simulink model "motor_channel"  (R2021a)
settings: configuration reference "motor_ctrl_config" (kept outside this file)
model workspace (MAT data in the model file):
  debounce_cnt = Simulink.Parameter
  debounce_cnt.Value = 4
  debounce_cnt.DataType = 'int16'
  debounce_cnt.Dimensions = [1 1]
  long_cnt = Simulink.Parameter
  long_cnt.Value = 6000
  long_cnt.DataType = 'int16'
  long_cnt.Dimensions = [1 1]
  longpress_cnt = Simulink.Parameter
  longpress_cnt.Value = 100
  longpress_cnt.DataType = 'int16'
  longpress_cnt.Dimensions = [1 1]
  short_cnt = Simulink.Parameter
  short_cnt.Value = 20
  short_cnt.DataType = 'int16'
  short_cnt.Dimensions = [1 1]
  transfer_cnt = Simulink.Parameter
  transfer_cnt.Value = 50
  transfer_cnt.DataType = 'int16'
  transfer_cnt.Dimensions = [1 1]
settings Model: DataDictionary=motor_ctrl_data.sldd  ParameterArgumentNames=debounce_cnt,long_cnt,longpress_cnt,short_cnt,transfer_cnt  OrderedModelArguments=off  Creator=Litao  LastModifiedBy=Litao
settings ConfigSetRef: SourceName=motor_ctrl_config

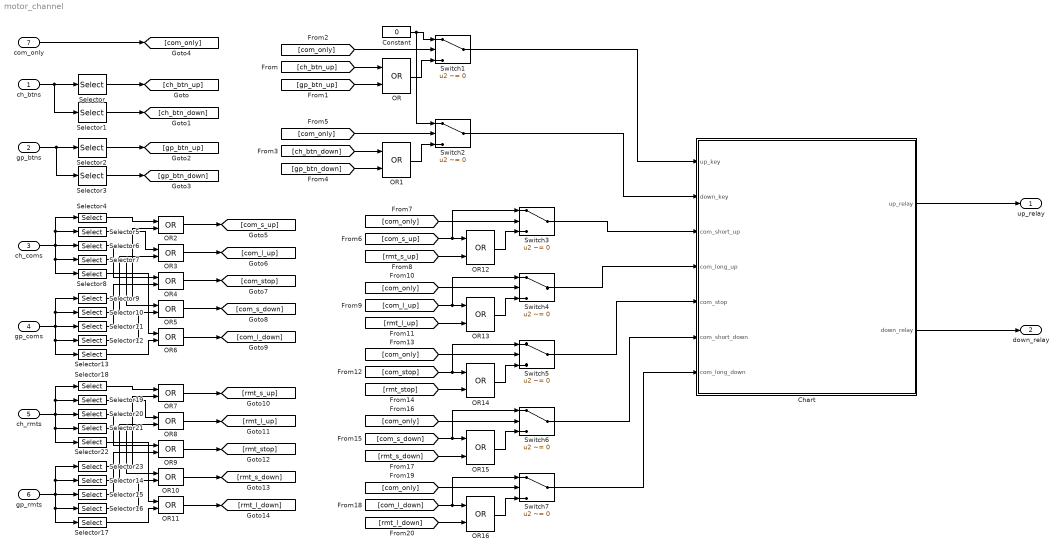
== system motor_channel ==
  ch_btns : Inport  OutMin=0  OutMax=1  OutDataTypeStr=int16  PortDimensions=2
  gp_btns : Inport  Port=2  OutMin=0  OutMax=1  OutDataTypeStr=int16  PortDimensions=2
  ch_coms : Inport  Port=3  OutMin=0  OutMax=1  OutDataTypeStr=int16  PortDimensions=5
  gp_coms : Inport  Port=4  OutMin=0  OutMax=1  OutDataTypeStr=int16  PortDimensions=5
  ch_rmts : Inport  Port=5  OutMin=0  OutMax=1  OutDataTypeStr=int16  PortDimensions=5
  gp_rmts : Inport  Port=6  OutMin=0  OutMax=1  OutDataTypeStr=int16  PortDimensions=5
  com_only : Inport  Port=7  OutMin=0  OutMax=1  OutDataTypeStr=int16  PortDimensions=1
  Chart : Stateflow chart
      settings: PortSchema="{\"entries\":[{\"content\":{\"sides\":[{\"content\":{\"connectorIds\":[\"In1\",\"In6\",\"In2\",\"In3\",\"In4\",\"In5\",\"In7\"]},\"type\":\"ConnectorPlacement.EquallySpacedRectSide\",\"uuid\":\"4c20fa99-1adf-4f22-ae93-c6186f058e35\"},{\"content\":{\"connectorIds\":[\"Out1\",\"Out2\"],\"side\":\"RIGHT\"},\"type\":\"ConnectorPlacement.EquallySpacedRectSide\",\"uuid\":\"7e4b4d75-813d-4fac-a5e7-b1188569f7b1\"},{\"content\":{\"connectorIds\":[],\"side\":\"TOP\"},\"type\":\"ConnectorPlacement.EquallySpacedRectSide\",\"uuid\":\"dfb94294-383a-4a0d-9cf2-9ac7874d8458\"}]},\"type\":\"ConnectorPlacement.EquallySpacedConnector\",\"uuid\":\"7d129faa-0032-4342-99de-de2067696b6a\"}],\"packageUris\":[\"http://schema.mathworks.com/mf0/Connector/R2020b\"],\"version\":\"1.0\"}"
  Constant : Constant  Value=0  OutDataTypeStr=int16
  OR{,1..16} (17 alike) : Logic  Operator=OR  AllPortsSameDT=off
  Selector : Selector  IndexMode=Zero-based  InputPortWidth=2  IndexOptions=Index vector (dialog)  Indices=[0]  OutputSizes=1
  Selector1 : Selector  IndexMode=Zero-based  InputPortWidth=2  IndexOptions=Index vector (dialog)  Indices=[1]  OutputSizes=1
  Selector{5,10,14,19} (4 alike) : Selector  IndexMode=Zero-based  InputPortWidth=5  IndexOptions=Index vector (dialog)  Indices=[1]  OutputSizes=1
  Selector{6,11,15,20} (4 alike) : Selector  IndexMode=Zero-based  InputPortWidth=5  IndexOptions=Index vector (dialog)  Indices=[2]  OutputSizes=1
  Selector{7,12,16,21} (4 alike) : Selector  IndexMode=Zero-based  InputPortWidth=5  IndexOptions=Index vector (dialog)  Indices=[3]  OutputSizes=1
  Selector{8,13,17,22} (4 alike) : Selector  IndexMode=Zero-based  InputPortWidth=5  IndexOptions=Index vector (dialog)  Indices=[4]  OutputSizes=1
  Selector{4,9,18,23} (4 alike) : Selector  IndexMode=Zero-based  InputPortWidth=5  IndexOptions=Index vector (dialog)  Indices=[0]  OutputSizes=1
  Selector2 : Selector  IndexMode=Zero-based  InputPortWidth=2  IndexOptions=Index vector (dialog)  Indices=[0]  OutputSizes=1
  Selector3 : Selector  IndexMode=Zero-based  InputPortWidth=2  IndexOptions=Index vector (dialog)  Indices=[1]  OutputSizes=1
  Switch{1..7} (7 alike) : Switch  Criteria=u2 ~= 0
  up_relay : Outport  OutMin=0  OutMax=1  OutDataTypeStr=int16  PortDimensions=1
  down_relay : Outport  Port=2  OutMin=0  OutMax=1  OutDataTypeStr=int16  PortDimensions=1
  wires:
  ch_btns/1 -> Selector1/1, Selector/1
  Selector/1 -> [ch_btn_up]
  Selector1/1 -> [ch_btn_down]
  Selector3/1 -> [gp_btn_down]
  Selector2/1 -> [gp_btn_up]
  gp_btns/1 -> Selector3/1, Selector2/1
  [ch_btn_up] -> OR/1
  [gp_btn_up] -> OR/2
  com_only/1 -> [com_only]
  [com_only] -> Switch1/2
  OR/1 -> Switch1/3
  ch_coms/1 -> Selector4/1, Selector5/1, Selector8/1, Selector7/1, Selector6/1
  Constant/1 -> Switch2/1, Switch1/1
  [com_only] -> Switch2/2
  [ch_btn_down] -> OR1/1
  OR1/1 -> Switch2/3
  [gp_btn_down] -> OR1/2
  gp_coms/1 -> Selector9/1, Selector10/1, Selector13/1, Selector12/1, Selector11/1
  Selector4/1 -> OR2/1
  Selector9/1 -> OR2/2
  Selector5/1 -> OR3/1
  Selector10/1 -> OR3/2
  Selector6/1 -> OR4/1
  Selector11/1 -> OR4/2
  Selector7/1 -> OR5/1
  Selector12/1 -> OR5/2
  Selector8/1 -> OR6/1
  Selector13/1 -> OR6/2
  OR2/1 -> [com_s_up]
  OR3/1 -> [com_l_up]
  OR4/1 -> [com_stop]
  OR5/1 -> [com_s_down]
  OR6/1 -> [com_l_down]
  Selector16/1 -> OR10/2
  OR8/1 -> [rmt_l_up]
  Selector20/1 -> OR9/1
  Selector21/1 -> OR10/1
  OR10/1 -> [rmt_s_down]
  Selector22/1 -> OR11/1
  OR7/1 -> [rmt_s_up]
  OR11/1 -> [rmt_l_down]
  Selector17/1 -> OR11/2
  Selector23/1 -> OR7/2
  Selector19/1 -> OR8/1
  Selector14/1 -> OR8/2
  ch_rmts/1 -> Selector18/1, Selector19/1, Selector22/1, Selector21/1, Selector20/1
  Selector15/1 -> OR9/2
  Selector18/1 -> OR7/1
  OR9/1 -> [rmt_stop]
  gp_rmts/1 -> Selector23/1, Selector14/1, Selector17/1, Selector16/1, Selector15/1
  OR12/1 -> Switch3/3
  [com_only] -> Switch3/2
  [rmt_s_up] -> OR12/2
  [com_s_up] -> Switch3/1, OR12/1
  [com_only] -> Switch4/2
  [rmt_l_up] -> OR13/2
  OR13/1 -> Switch4/3
  [com_l_up] -> Switch4/1, OR13/1
  [com_only] -> Switch5/2
  [rmt_stop] -> OR14/2
  OR14/1 -> Switch5/3
  [com_stop] -> Switch5/1, OR14/1
  [com_only] -> Switch6/2
  [rmt_s_down] -> OR15/2
  OR15/1 -> Switch6/3
  [com_s_down] -> Switch6/1, OR15/1
  [com_only] -> Switch7/2
  [rmt_l_down] -> OR16/2
  OR16/1 -> Switch7/3
  [com_l_down] -> Switch7/1, OR16/1
  Switch1/1 -> Chart/1(up_key)
  Switch2/1 -> Chart/6(down_key)
  Switch3/1 -> Chart/2(com_short_up)
  Switch4/1 -> Chart/3(com_long_up)
  Switch5/1 -> Chart/4(com_stop)
  Switch6/1 -> Chart/5(com_short_down)
  Switch7/1 -> Chart/7(com_long_down)
  Chart/1(up_relay) -> up_relay/1
  Chart/2(down_relay) -> down_relay/1

== stateflow chart motor_channel/Chart ==
  state MOTOR_CTRL
    state COM_CMD [parallel]
      settings: executionOrder=1
      state SHORT_DOWN
        en: send(short_down_event,MOTOR)
      state IDLE
      state SHORT_UP
        en: send(short_up_event,MOTOR)
      state LONG_DOWN
        en: send(long_down_event,MOTOR)
      state LONG_UP
        en: send(long_up_event,MOTOR)
      state STOP
        en: send(stop_event,MOTOR)
      (default) -> MOTOR_CTRL.COM_CMD.IDLE
      MOTOR_CTRL.COM_CMD.IDLE -> MOTOR_CTRL.COM_CMD.SHORT_UP [order 3] : [com_short_up==1]
      MOTOR_CTRL.COM_CMD.IDLE -> MOTOR_CTRL.COM_CMD.SHORT_DOWN [order 5] : [com_short_down==1]
      MOTOR_CTRL.COM_CMD.SHORT_DOWN -> MOTOR_CTRL.COM_CMD.IDLE : [after(short_cnt,tick)]
      MOTOR_CTRL.COM_CMD.SHORT_UP -> MOTOR_CTRL.COM_CMD.IDLE : [after(short_cnt,tick)]
      MOTOR_CTRL.COM_CMD.IDLE -> MOTOR_CTRL.COM_CMD.LONG_DOWN [order 1] : [com_long_down==1]
      MOTOR_CTRL.COM_CMD.LONG_DOWN -> MOTOR_CTRL.COM_CMD.IDLE : [after(short_cnt,tick)]
      MOTOR_CTRL.COM_CMD.IDLE -> STOP [order 2] : [com_stop==1]
      STOP -> MOTOR_CTRL.COM_CMD.IDLE : [after(short_cnt,tick)]
      MOTOR_CTRL.COM_CMD.LONG_UP -> MOTOR_CTRL.COM_CMD.IDLE : [after(short_cnt,tick)]
      MOTOR_CTRL.COM_CMD.IDLE -> MOTOR_CTRL.COM_CMD.LONG_UP [order 4] : [com_long_up==1]
    state KEY_CMD [parallel]
      settings: executionOrder=2
      state DOWN_KEY_PRESSED
        state DOWN_CLICK
        state DOWN_DEBOUNCE
        state DOWN_LONGPRESS
          en: send(down_key_long_press,MOTOR)
        (default) -> DOWN_DEBOUNCE
        DOWN_DEBOUNCE -> DOWN_CLICK [order 1] : [after(debounce_cnt,tick)]
        DOWN_CLICK -> DOWN_LONGPRESS [order 2] : [after(longpress_cnt,tick)]
      state IDLE
      state UP_KEY_PRESSED
        state UP_DEBOUNCE
        state UP_CLICK
        state UP_LONGPRESS
          en: send(up_key_long_press,MOTOR)
        (default) -> UP_DEBOUNCE
        UP_DEBOUNCE -> UP_CLICK [order 1] : [after(debounce_cnt,tick)]
        UP_CLICK -> UP_LONGPRESS [order 2] : [after(longpress_cnt,tick)]
      (default) -> MOTOR_CTRL.KEY_CMD.IDLE
      MOTOR_CTRL.KEY_CMD.IDLE -> UP_KEY_PRESSED [order 1] : [up_key==1]
      MOTOR_CTRL.KEY_CMD.IDLE -> DOWN_DEBOUNCE [order 2] : [down_key==1]
      UP_DEBOUNCE -> MOTOR_CTRL.KEY_CMD.IDLE [order 2] : [up_key~=1]
      DOWN_DEBOUNCE -> MOTOR_CTRL.KEY_CMD.IDLE [order 2] : [down_key~=1]
      UP_CLICK -> MOTOR_CTRL.KEY_CMD.IDLE [order 1] : [up_key~=1]{send(up_key_click,MOTOR)}
      DOWN_CLICK -> MOTOR_CTRL.KEY_CMD.IDLE [order 1] : [down_key~=1]{send(down_key_click, MOTOR)}
      UP_LONGPRESS -> MOTOR_CTRL.KEY_CMD.IDLE : [up_key~=1]
      DOWN_LONGPRESS -> MOTOR_CTRL.KEY_CMD.IDLE : [down_key~=1]
    state MOTOR [parallel]
      settings: executionOrder=3
      state SHORT_DOWN
        en: down_relay=1;
        ex: down_relay=0;
      state OFF
      state SHORT_UP
        en: up_relay=1;
        ex: up_relay=0;
      state LONG_DOWN
        en: down_relay=1;
        ex: down_relay=0;
      state LONG_UP
        en: up_relay=1;
        ex: up_relay=0;
      state UP_TO_LONGDOWN
      state DOWN_TO_LONGUP
      (default) -> OFF
      OFF -> MOTOR_CTRL.MOTOR.SHORT_DOWN [order 3] : [down_key_click || short_down_event]
      OFF -> MOTOR_CTRL.MOTOR.SHORT_UP [order 1] : [up_key_click || short_up_event]
      MOTOR_CTRL.MOTOR.SHORT_UP -> OFF : [after(short_cnt,tick)]
      MOTOR_CTRL.MOTOR.SHORT_DOWN -> OFF : [after(short_cnt,tick)]
      OFF -> MOTOR_CTRL.MOTOR.LONG_UP [order 2] : [up_key_long_press || long_up_event]
      OFF -> MOTOR_CTRL.MOTOR.LONG_DOWN [order 4] : [down_key_long_press || long_down_event]
      MOTOR_CTRL.MOTOR.LONG_UP -> OFF [order 2] : [up_key_click || down_key_click ||stop_event ||after(long_cnt,tick)]
      MOTOR_CTRL.MOTOR.LONG_DOWN -> OFF [order 1] : [down_key_click || up_key_click || stop_event ||after(long_cnt,tick)]
      UP_TO_LONGDOWN -> MOTOR_CTRL.MOTOR.LONG_DOWN : [after(transfer_cnt, tick)]
      MOTOR_CTRL.MOTOR.LONG_UP -> UP_TO_LONGDOWN [order 1] : [down_key_long_press || long_down_event]
      MOTOR_CTRL.MOTOR.LONG_DOWN -> DOWN_TO_LONGUP [order 2] : [up_key_long_press || long_up_event]
      DOWN_TO_LONGUP -> MOTOR_CTRL.MOTOR.LONG_UP : [after(transfer_cnt, tick)]
  (default) -> MOTOR_CTRL
  data: up_key input; com_short_up input; com_long_up input; com_stop input; com_short_down input; down_key input; com_long_down input; up_relay output int16; down_relay output int16; debounce_cnt parameter size=1; longpress_cnt parameter size=1; transfer_cnt parameter; short_cnt parameter; long_cnt parameter
  events: long_down_event local FUNCTION_CALL_EVENT; long_up_event local FUNCTION_CALL_EVENT; short_down_event local FUNCTION_CALL_EVENT; short_up_event local FUNCTION_CALL_EVENT; stop_event local FUNCTION_CALL_EVENT; down_key_click local FUNCTION_CALL_EVENT; down_key_long_press local FUNCTION_CALL_EVENT; up_key_click local FUNCTION_CALL_EVENT; up_key_long_press local FUNCTION_CALL_EVENT
